simulink model "Torque Vectoring"  (R2023b)
settings: Solver=VariableStepAuto  StartTime=0.0  StopTime=10.0  RelTol=1e-3
model workspace (MAT data in the model file):
  Bx = 10
  By = 10
  Cd = 0.2
  Cx = 1.9
  Cy = 1.9
  Ex = 0.97
  Ey = 0.97
  Izz = 600
  Ki = 1
  Kp = 1
  Ku = 1
  Re = 0.25
  Ts = 0.01
  g = 9.8
  h = 0.3
  k = 100
  l = 2.25
  lf = 0.78
  lr = 0.78
  m = 300
  mu_x = 0.3
  mu_y = 0.2
  rho = 8
  s = 1
libraries: slpidlib x1
settings Model: Creator=Anand Chutani  LastModifiedBy=Anand Chutani
settings DebuggingCC: AlgebraicLoopMsg=none

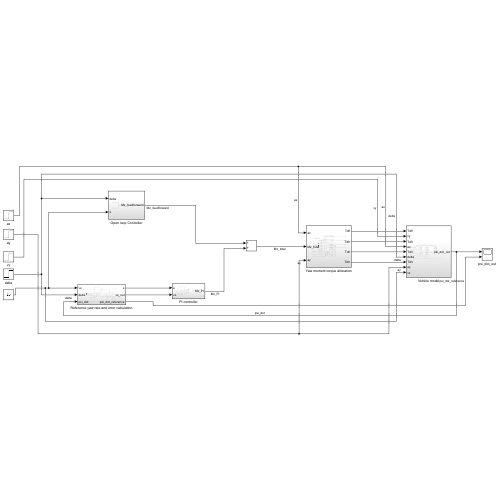
[thumbnail: Simulink's stored preview of the top-level diagram]
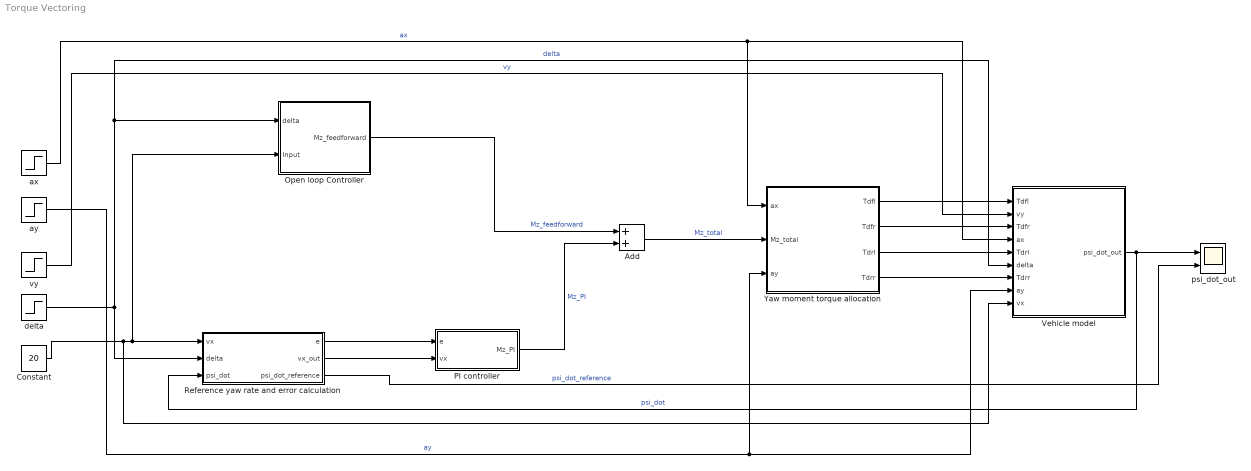
== system Torque Vectoring ==
  Add : Sum
  Constant : Constant  Value=20
  Open loop Controller : Subsystem
  PI controller : Subsystem
  Reference yaw rate and error calculation : Subsystem
  Vehicle model : Subsystem
  Yaw moment torque allocation : Subsystem
  ax : Step  Before=1  After=3  SampleTime=0
  ay : Step  Before=1  After=5  SampleTime=0
  delta : Step  Before=1  After=4  SampleTime=0
  psi_dot_out : Scope  NumInputPorts=2
  vy : Step  Before=12  After=14  SampleTime=0
  wires:
  Add/1 -> Yaw moment torque allocation/2(Mz_total)  "Mz_total"
  Yaw moment torque allocation/1(Tdfl) -> Vehicle model/1(Tdfl)
  Yaw moment torque allocation/2(Tdfr) -> Vehicle model/3(Tdfr)
  Yaw moment torque allocation/3(Tdrl) -> Vehicle model/5(Tdrl)
  Yaw moment torque allocation/4(Tdrr) -> Vehicle model/7(Tdrr)
  delta/1 -> Vehicle model/6(delta), Open loop Controller/1(delta), Reference yaw rate and error calculation/2(delta)  "delta"
  Vehicle model/1(psi_dot_out) -> Reference yaw rate and error calculation/3(psi_dot), psi_dot_out/1  "psi_dot"
  ax/1 -> Yaw moment torque allocation/1(ax), Vehicle model/4(ax)  "ax"
  ay/1 -> Yaw moment torque allocation/3(ay), Vehicle model/8(ay)  "ay"
  vy/1 -> Vehicle model/2(vy)  "vy"
  Reference yaw rate and error calculation/3(psi_dot_reference) -> psi_dot_out/2  "psi_dot_reference"
  Reference yaw rate and error calculation/1(e) -> PI controller/1(e)
  PI controller/1(Mz_PI) -> Add/2  "Mz_PI"
  Open loop Controller/1(Mz_feedforward) -> Add/1  "Mz_feedforward"
  Reference yaw rate and error calculation/2(vx_out) -> PI controller/2(vx)
  Constant/1 -> Vehicle model/9(vx), Open loop Controller/2(Input), Reference yaw rate and error calculation/1(vx)

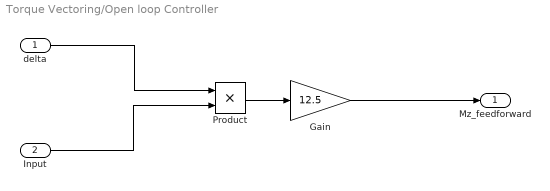
== system Torque Vectoring/Open loop Controller ==
  delta : Inport
  Input : Inport  Port=2
  Gain : Gain  Gain=12.5
  Product : Product
  Mz_feedforward : Outport
  wires:
  Gain/1 -> Mz_feedforward/1
  delta/1 -> Product/1
  Input/1 -> Product/2
  Product/1 -> Gain/1

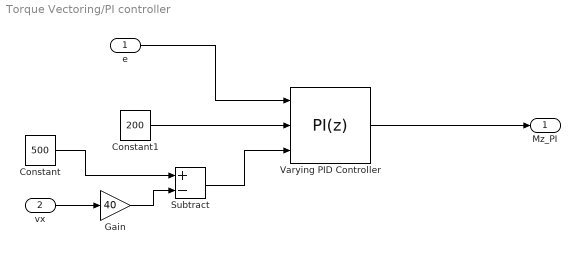
== system Torque Vectoring/PI controller ==
  e : Inport
  vx : Inport  Port=2
  Constant : Constant  Value=500
  Constant1 : Constant  Value=200
  Gain : Gain  Gain=40
  Subtract : Sum  Inputs=+-
  Varying PID Controller : slpidlib/PID Controller  Controller=PI  Form=Parallel  TimeDomain=Discrete-time  UseExternalTs=off  SampleTime=-1  IntegratorMethod=Forward Euler  FilterMethod=Forward Euler  ControllerParametersSource=external  P=1  I=1  UseKiTs=off  D=0  N=100  UseFilter=on  TunerSelectOption=Transfer Function Based (PID Tuner App)  InitialConditionSource=internal  InitialConditionForIntegrator=0  InitialConditionForFilter=0  DifferentiatorICPrevScaledInput=0  ExternalReset=none  TrackingMode=off  Kt=1  LimitOutput=off  SatLimitsSource=internal  UpperSaturationLimit=inf  LowerSaturationLimit=-inf  LinearizeAsGain=on  AntiWindupMode=none  Kb=1  LimitIntegrator=off  UpperIntegratorSaturationLimit=inf  LowerIntegratorSaturationLimit=-inf  POutMin=[]  POutMax=[]  IOutMin=[]  IOutMax=[]  DOutMin=[]  DOutMax=[]  NOutMin=[]  NOutMax=[]  SumOutMin=[]  SumOutMax=[]  SaturationOutMin=[]  SaturationOutMax=[]  PParamMin=[]  PParamMax=[]  IParamMin=[]  IParamMax=[]  DParamMin=[]  DParamMax=[]  NParamMin=[]  NParamMax=[]  KbParamMin=[]  KbParamMax=[]  KtParamMin=[]  KtParamMax=[]  KbOutMin=[]  KbOutMax=[]  KtOutMin=[]  KtOutMax=[]  IntegratorOutMin=[]  IntegratorOutMax=[]  FilterOutMin=[]  FilterOutMax=[]  SumI1OutMin=[]  SumI1OutMax=[]  SumI2OutMin=[]  SumI2OutMax=[]  SumI3OutMin=[]  SumI3OutMax=[]  SumI4OutMin=[]  SumI4OutMax=[]  SumDOutMin=[]  SumDOutMax=[]  DifferentiatorOutMin=[]  DifferentiatorOutMax=[]  FilterDiffOutCoefMin=[]  FilterDiffOutCoefMax=[]  ReciprocalOutMin=[]  ReciprocalOutMax=[]  SumDenOutMin=[]  SumDenOutMax=[]  SumNumOutMin=[]  SumNumOutMax=[]  DivideOutMin=[]  DivideOutMax=[]  UdiffTsProdOutMin=[]  UdiffTsProdOutMax=[]  NTsProdOutMin=[]  NTsProdOutMax=[]  UintegralTsProdOutMin=[]  UintegralTsProdOutMax=[]  UngainTsProdOutMin=[]  UngainTsProdOutMax=[]  ClampingZeroOutDataTypeStr=Inherit: Inherit via back propagation  ClampingZeroOutMin=[]  ClampingZeroOutMax=[]  FilterDenConstantOutDataTypeStr=Inherit: Inherit via back propagation  FilterDenConstantOutMin=[]  FilterDenConstantOutMax=[]  PCopyOutDataTypeStr=Inherit: Inherit via back propagation  PCopyOutMin=[]  PCopyOutMax=[]  NCopyOutDataTypeStr=Inherit: Inherit via back propagation  NCopyOutMin=[]  NCopyOutMax=[]  IntegratorContinuousStateAttributes=''  IntegratorStateMustResolveToSignalObject=off  IntegratorRTWStateStorageClass=Auto  FilterContinuousStateAttributes=''  FilterStateMustResolveToSignalObject=off  FilterRTWStateStorageClass=Auto  ParallelPVariant=ExternalParameters  IdealPVariant=Disabled  IVariant=ExternalParameters  DVariant=Disabled  IntegratorVariant=Discrete  SatVariant=Disabled  AWVariant=Passthrough  PCopyVariant=Disabled  TRVariant=Disabled  FdbkBlocksVariant=Forward  IdealPFdbkVariant=Disabled  SatFdbkVariant=Disabled  DerivativeFilterVariant=Disabled  NVariant=Disabled  NCopyVariant=Disabled_SignalSpec  FilterICVariant=Disabled  IntegratorICVariant=InternalICs  ExternalResetVariant=Disabled  TRSumVariant=Passthrough  SumFdbkVariant=Disabled  SumVariant=Sum_PI  TsampFilterVariant=InternalTs  TsampNgainVariant=Passthrough  TsampIntegralVariant=Disabled_SignalSpec  ExternalSaturationOutDataTypeStr=Inherit: Same as second input
      settings: LibrarySourceBlock=cstblocks/Linear Parameter Varying/Varying PID Controller
  Mz_PI : Outport
  wires:
  Varying PID Controller/1 -> Mz_PI/1
  vx/1 -> Gain/1
  e/1 -> Varying PID Controller/1
  Constant/1 -> Subtract/1
  Subtract/1 -> Varying PID Controller/3
  Constant1/1 -> Varying PID Controller/2
  Gain/1 -> Subtract/2

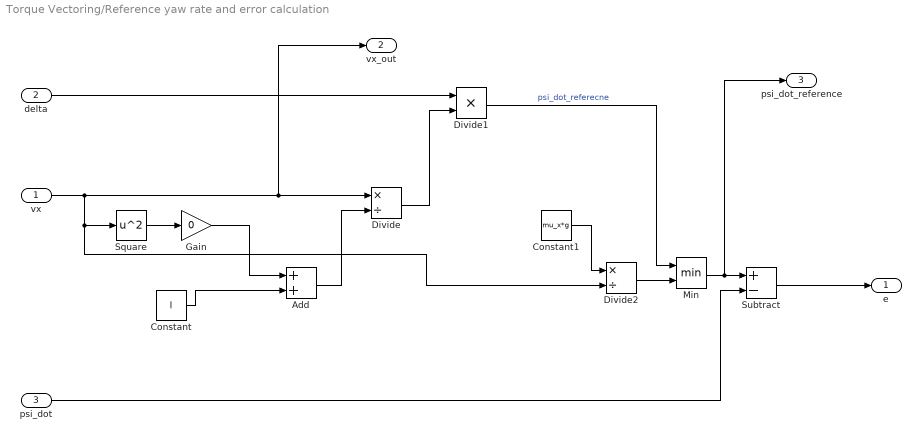
== system Torque Vectoring/Reference yaw rate and error calculation ==
  vx : Inport
  delta : Inport  Port=2
  psi_dot : Inport  Port=3
  Add : Sum
  Constant : Constant  Value=l
  Constant1 : Constant  Value=mu_x*g
  Divide : Product  Inputs=*/
  Divide1 : Product  Inputs=**
  Divide2 : Product  Inputs=*/
  Gain : Gain  Gain=0
  Min : MinMax  Inputs=2
  Square : Math  Operator=square
  Subtract : Sum  Inputs=+-
  e : Outport
  vx_out : Outport  Port=2
  psi_dot_reference : Outport  Port=3
  wires:
  vx/1 -> vx_out/1, Divide/1, Divide2/2, Square/1
  Square/1 -> Gain/1
  Gain/1 -> Add/1
  Constant/1 -> Add/2
  Add/1 -> Divide/2
  delta/1 -> Divide1/1
  Divide/1 -> Divide1/2
  Divide1/1 -> Min/1  "psi_dot_referecne"
  psi_dot/1 -> Subtract/2
  Subtract/1 -> e/1
  Constant1/1 -> Divide2/1
  Divide2/1 -> Min/2
  Min/1 -> psi_dot_reference/1, Subtract/1

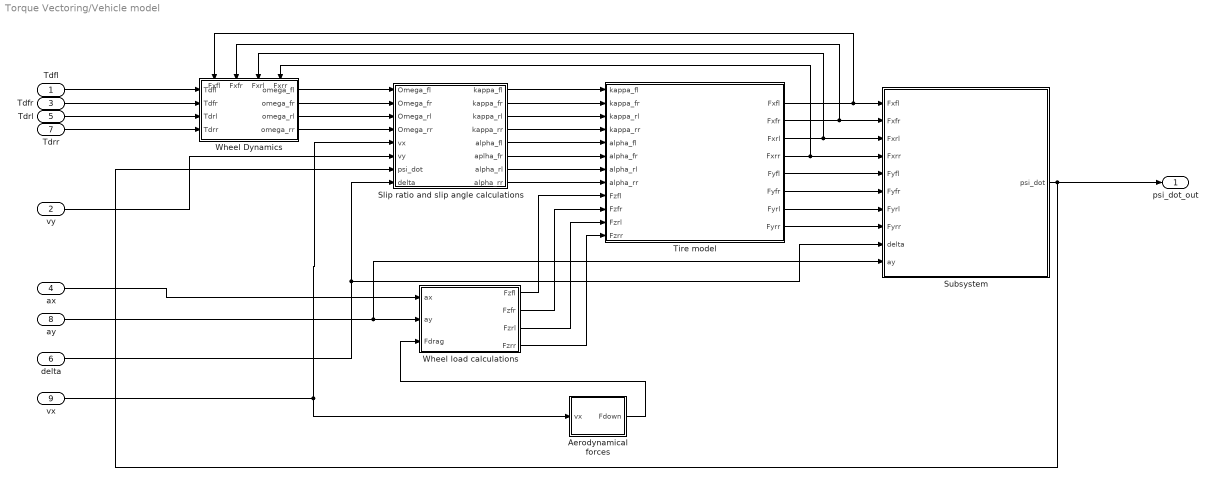
== system Torque Vectoring/Vehicle model ==
  Tdfl : Inport
  vy : Inport  Port=2
  Tdfr : Inport  Port=3
  ax : Inport  Port=4
  Tdrl : Inport  Port=5
  delta : Inport  Port=6
  Tdrr : Inport  Port=7
  ay : Inport  Port=8
  vx : Inport  Port=9
  Aerodynamical forces : Subsystem
  Slip ratio and slip angle calculations : Subsystem
  Subsystem : Subsystem
  Tire model : Subsystem
  Wheel Dynamics : Subsystem
      settings: PortSchema="{\"entries\":[{\"content\":{\"sides\":[{\"content\":{\"connectorIds\":[\"In1\",\"In2\",\"In3\",\"In4\"]},\"type\":\"ConnectorPlacement.EquallySpacedRectSide\",\"uuid\":\"cf3d01e9-74dd-45bb-b04b-f5977a1fd43e\"},{\"content\":{\"connectorIds\":[\"Out1\",\"Out2\",\"Out3\",\"Out4\"],\"side\":\"RIGHT\"},\"type\":\"ConnectorPlacement.EquallySpacedRectSide\",\"uuid\":\"48e33519-fc03-4ace-b300-f3df5174e3b2\"},{\"content\":{\"connectorIds\":[\"In5\",\"In6\",\"In7\",\"In8\"],\"side\":\"TOP\"},\"type\":\"ConnectorPlacement.EquallySpacedRectSide\",\"uuid\":\"343d2f22-4e97-404d-bc1a-e31503635e2d\"}]},\"type\":\"ConnectorPlacement.EquallySpacedConnector\",\"uuid\":\"a3e340ec-438c-437e-9241-e2a33ee22be6\"}],\"packageUris\":[\"http://schema.mathworks.com/mf0/Connector/R2020b\"],\"version\":\"1.0\"}"
  Wheel load calculations : Subsystem
  psi_dot_out : Outport
  wires:
  Wheel Dynamics/1(omega_fl) -> Slip ratio and slip angle calculations/1(Omega_fl)
  Wheel Dynamics/2(omega_fr) -> Slip ratio and slip angle calculations/2(Omega_fr)
  Wheel Dynamics/3(omega_rl) -> Slip ratio and slip angle calculations/3(Omega_rl)
  Wheel Dynamics/4(omega_rr) -> Slip ratio and slip angle calculations/4(Omega_rr)
  vy/1 -> Slip ratio and slip angle calculations/6(vy)
  delta/1 -> Slip ratio and slip angle calculations/8(delta), Subsystem/9(delta)
  Aerodynamical forces/1(Fdown) -> Wheel load calculations/3(Fdrag)
  Slip ratio and slip angle calculations/1(kappa_fl) -> Tire model/1(kappa_fl)
  Slip ratio and slip angle calculations/2(kappa_fr) -> Tire model/2(kappa_fr)
  Slip ratio and slip angle calculations/3(kappa_rl) -> Tire model/3(kappa_rl)
  Slip ratio and slip angle calculations/4(kappa_rr) -> Tire model/4(kappa_rr)
  Slip ratio and slip angle calculations/5(alpha_fl) -> Tire model/5(alpha_fl)
  Slip ratio and slip angle calculations/6(aplha_fr) -> Tire model/6(alpha_fr)
  Slip ratio and slip angle calculations/7(alpha_rl) -> Tire model/7(alpha_rl)
  Slip ratio and slip angle calculations/8(alpha_rr) -> Tire model/8(alpha_rr)
  Wheel load calculations/1(Fzfl) -> Tire model/9(Fzfl)
  Wheel load calculations/2(Fzfr) -> Tire model/10(Fzfr)
  Wheel load calculations/3(Fzrl) -> Tire model/11(Fzrl)
  Wheel load calculations/4(Fzrr) -> Tire model/12(Fzrr)
  Tire model/1(Fxfl) -> Wheel Dynamics/5(Fxfl), Subsystem/1(Fxfl)
  Tire model/2(Fxfr) -> Subsystem/2(Fxfr), Wheel Dynamics/6(Fxfr)
  Tire model/3(Fxrl) -> Wheel Dynamics/7(Fxrl), Subsystem/3(Fxrl)
  Tire model/4(Fxrr) -> Subsystem/4(Fxrr), Wheel Dynamics/8(Fxrr)
  Tire model/5(Fyfl) -> Subsystem/5(Fyfl)
  Tire model/6(Fyfr) -> Subsystem/6(Fyfr)
  Tire model/7(Fyrl) -> Subsystem/7(Fyrl)
  Tire model/8(Fyrr) -> Subsystem/8(Fyrr)
  ay/1 -> Wheel load calculations/2(ay), Subsystem/10(ay)
  ax/1 -> Wheel load calculations/1(ax)
  Subsystem/1(psi_dot) -> psi_dot_out/1, Slip ratio and slip angle calculations/7(psi_dot)
  Tdfl/1 -> Wheel Dynamics/1(Tdfl)
  Tdfr/1 -> Wheel Dynamics/2(Tdfr)
  Tdrl/1 -> Wheel Dynamics/3(Tdrl)
  Tdrr/1 -> Wheel Dynamics/4(Tdrr)
  vx/1 -> Slip ratio and slip angle calculations/5(vx), Aerodynamical forces/1(vx)

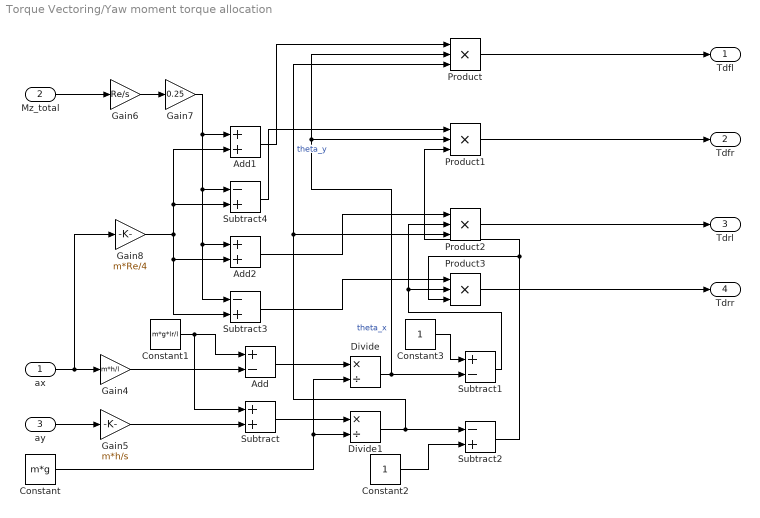
== system Torque Vectoring/Yaw moment torque allocation ==
  ax : Inport
  Mz_total : Inport  Port=2
  ay : Inport  Port=3
  Add : Sum  Inputs=+-
  Add1 : Sum
  Add2 : Sum
  Constant : Constant  Value=m*g
  Constant1 : Constant  Value=m*g*lr/l
  Constant2 : Constant
  Constant3 : Constant
  Divide : Product  Inputs=*/
  Divide1 : Product  Inputs=*/
  Gain4 : Gain  Gain=m*h/l
  Gain5 : Gain  Gain=m*h/s
  Gain6 : Gain  Gain=Re/s
  Gain7 : Gain  Gain=0.25
  Gain8 : Gain  Gain=m*Re/4
  Product{,1..3} (4 alike) : Product  Inputs=3
  Subtract : Sum
  Subtract1 : Sum  Inputs=+-
  Subtract2 : Sum  Inputs=-+
  Subtract3 : Sum  Inputs=-+
  Subtract4 : Sum  Inputs=-+
  Tdfl : Outport
  Tdfr : Outport  Port=2
  Tdrl : Outport  Port=3
  Tdrr : Outport  Port=4
  wires:
  ax/1 -> Gain8/1, Gain4/1
  ay/1 -> Gain5/1
  Constant1/1 -> Subtract/1, Add/1
  Gain4/1 -> Add/2
  Add/1 -> Divide/1
  Constant/1 -> Divide1/2, Divide/2
  Divide/1 -> Subtract1/2, Product1/2, Product/2  "theta_x"
  Gain5/1 -> Subtract/2
  Subtract/1 -> Divide1/1
  Divide1/1 -> Subtract2/1, Product/3, Product2/3  "theta_y"
  Constant2/1 -> Subtract2/2
  Constant3/1 -> Subtract1/1
  Subtract2/1 -> Product1/3, Product3/3
  Subtract1/1 -> Product3/2, Product2/2
  Mz_total/1 -> Gain6/1
  Gain6/1 -> Gain7/1
  Gain7/1 -> Subtract4/1, Subtract3/1, Add2/1, Add1/1
  Add1/1 -> Product/1
  Subtract4/1 -> Product1/1
  Add2/1 -> Product2/1
  Subtract3/1 -> Product3/1
  Product/1 -> Tdfl/1
  Product1/1 -> Tdfr/1
  Product2/1 -> Tdrl/1
  Product3/1 -> Tdrr/1
  Gain8/1 -> Subtract3/2, Add2/2, Subtract4/2, Add1/2

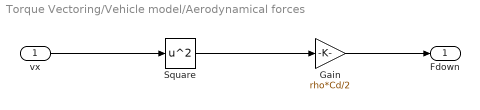
== system Torque Vectoring/Vehicle model/Aerodynamical forces ==
  vx : Inport
  Gain : Gain  Gain=rho*Cd/2
  Square : Math  Operator=square
  Fdown : Outport
  wires:
  vx/1 -> Square/1
  Gain/1 -> Fdown/1
  Square/1 -> Gain/1

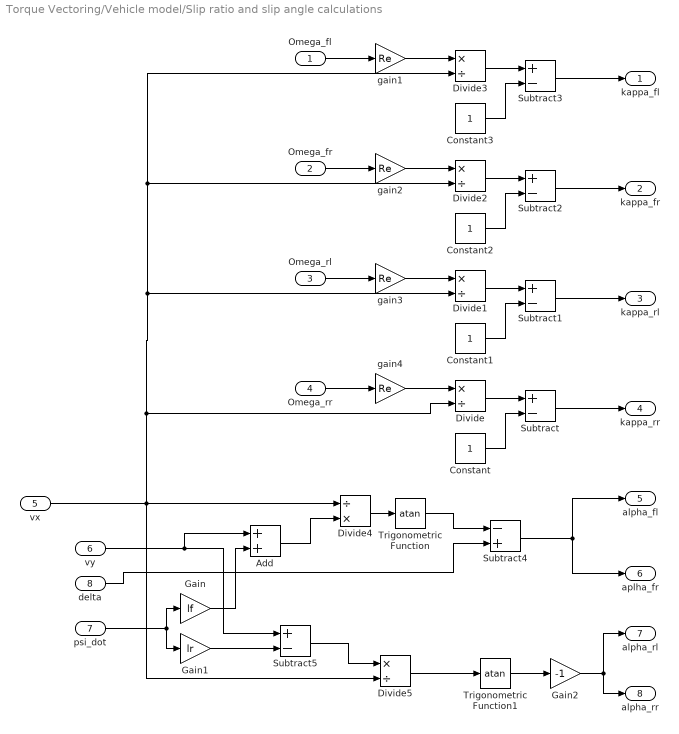
== system Torque Vectoring/Vehicle model/Slip ratio and slip angle calculations ==
  Omega_fl : Inport
  Omega_fr : Inport  Port=2
  Omega_rl : Inport  Port=3
  Omega_rr : Inport  Port=4
  vx : Inport  Port=5
  vy : Inport  Port=6
  psi_dot : Inport  Port=7
  delta : Inport  Port=8
  Add : Sum
  Constant{,1..3} (4 alike) : Constant
  Divide{,1..3,5} (5 alike) : Product  Inputs=*/
  Divide4 : Product  Inputs=/*
  Gain : Gain  Gain=lf
  Gain1 : Gain  Gain=lr
  Gain2 : Gain  Gain=-1
  Subtract{,1..3,5} (5 alike) : Sum  Inputs=+-
  Subtract4 : Sum  Inputs=-+
  Trigonometric Function : Trigonometry  Operator=atan
  Trigonometric Function1 : Trigonometry  Operator=atan
  gain{1..4} (4 alike) : Gain  Gain=Re
  kappa_fl : Outport
  kappa_fr : Outport  Port=2
  kappa_rl : Outport  Port=3
  kappa_rr : Outport  Port=4
  alpha_fl : Outport  Port=5
  aplha_fr : Outport  Port=6
  alpha_rl : Outport  Port=7
  alpha_rr : Outport  Port=8
  wires:
  Omega_rr/1 -> gain4/1
  gain4/1 -> Divide/1
  Divide/1 -> Subtract/1
  Constant/1 -> Subtract/2
  Subtract/1 -> kappa_rr/1
  Subtract1/1 -> kappa_rl/1
  gain3/1 -> Divide1/1
  Constant1/1 -> Subtract1/2
  Omega_rl/1 -> gain3/1
  Divide1/1 -> Subtract1/1
  Subtract2/1 -> kappa_fr/1
  gain2/1 -> Divide2/1
  Constant2/1 -> Subtract2/2
  Omega_fr/1 -> gain2/1
  Divide2/1 -> Subtract2/1
  Subtract3/1 -> kappa_fl/1
  gain1/1 -> Divide3/1
  Constant3/1 -> Subtract3/2
  Omega_fl/1 -> gain1/1
  Divide3/1 -> Subtract3/1
  vy/1 -> Subtract5/1, Add/1
  psi_dot/1 -> Gain1/1, Gain/1
  Gain/1 -> Add/2
  Add/1 -> Divide4/2
  Divide4/1 -> Trigonometric Function/1
  delta/1 -> Subtract4/2
  Trigonometric Function/1 -> Subtract4/1
  Subtract4/1 -> aplha_fr/1, alpha_fl/1
  Gain1/1 -> Subtract5/2
  Subtract5/1 -> Divide5/1
  Trigonometric Function1/1 -> Gain2/1
  Gain2/1 -> alpha_rr/1, alpha_rl/1
  Divide5/1 -> Trigonometric Function1/1
  vx/1 -> Divide3/2, Divide2/2, Divide1/2, Divide/2, Divide4/1, Divide5/2

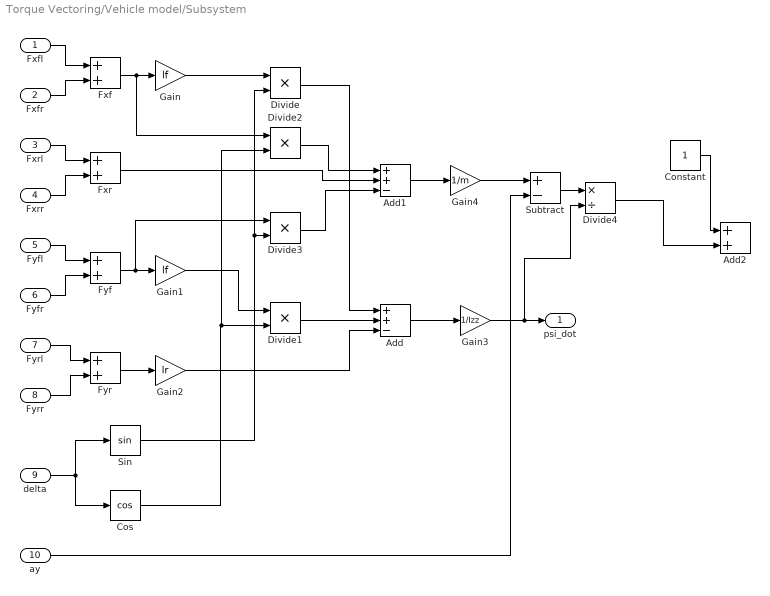
== system Torque Vectoring/Vehicle model/Subsystem ==
  Fxfl : Inport
  Fxfr : Inport  Port=2
  Fxrl : Inport  Port=3
  Fxrr : Inport  Port=4
  Fyfl : Inport  Port=5
  Fyfr : Inport  Port=6
  Fyrl : Inport  Port=7
  Fyrr : Inport  Port=8
  delta : Inport  Port=9
  ay : Inport  Port=10
  Add : Sum  Inputs=++-
  Add1 : Sum  Inputs=++-
  Add2 : Sum
  Constant : Constant
  Cos : Trigonometry  Operator=cos
  Divide{,1..3} (4 alike) : Product  Inputs=**
  Divide4 : Product  Inputs=*/
  Fxf : Sum
  Fxr : Sum
  Fyf : Sum
  Fyr : Sum
  Gain : Gain  Gain=lf
  Gain1 : Gain  Gain=lf
  Gain2 : Gain  Gain=lr
  Gain3 : Gain  Gain=1/Izz
  Gain4 : Gain  Gain=1/m
  Sin : Trigonometry
  Subtract : Sum  Inputs=+-
  psi_dot : Outport
  wires:
  Fxfl/1 -> Fxf/1
  Fxfr/1 -> Fxf/2
  Fxrl/1 -> Fxr/1
  Fxrr/1 -> Fxr/2
  Fyfl/1 -> Fyf/1
  Fyfr/1 -> Fyf/2
  Fyrl/1 -> Fyr/1
  Fyrr/1 -> Fyr/2
  Fxf/1 -> Divide2/1, Gain/1
  delta/1 -> Cos/1, Sin/1
  Sin/1 -> Divide3/2, Divide/2
  Gain/1 -> Divide/1
  Fyf/1 -> Divide3/1, Gain1/1
  Gain1/1 -> Divide1/1
  Cos/1 -> Divide2/2, Divide1/2
  Fyr/1 -> Gain2/1
  Divide/1 -> Add/1
  Divide1/1 -> Add/2
  Gain2/1 -> Add/3
  Add/1 -> Gain3/1
  Gain3/1 -> Divide4/2, psi_dot/1
  Divide2/1 -> Add1/1
  Fxr/1 -> Add1/2
  Divide3/1 -> Add1/3
  Add1/1 -> Gain4/1
  Gain4/1 -> Subtract/1
  ay/1 -> Subtract/2
  Subtract/1 -> Divide4/1
  Divide4/1 -> Add2/2
  Constant/1 -> Add2/1

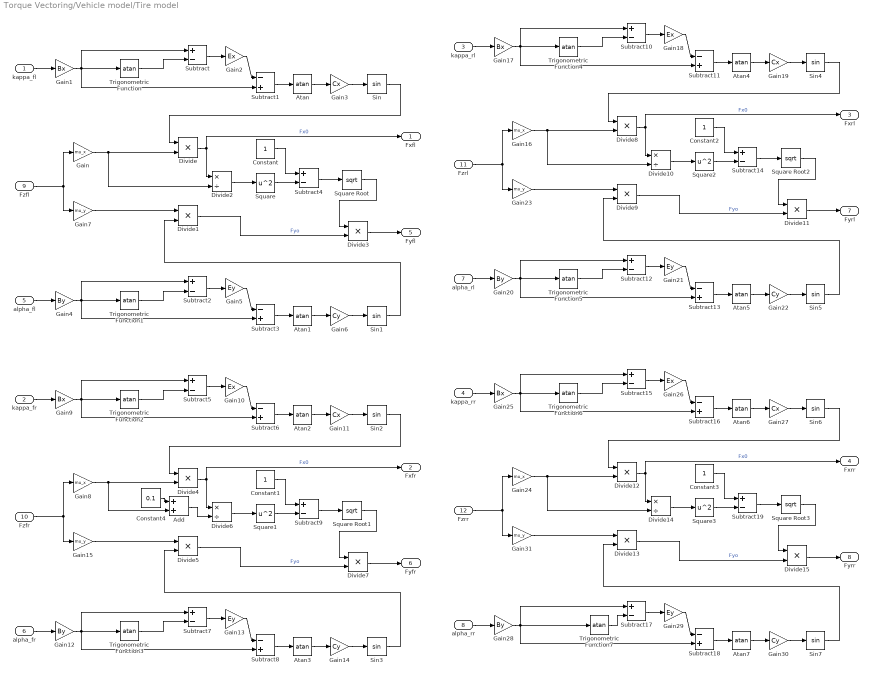
== system Torque Vectoring/Vehicle model/Tire model ==
  kappa_fl : Inport
  kappa_fr : Inport  Port=2
  kappa_rl : Inport  Port=3
  kappa_rr : Inport  Port=4
  alpha_fl : Inport  Port=5
  alpha_fr : Inport  Port=6
  alpha_rl : Inport  Port=7
  alpha_rr : Inport  Port=8
  Fzfl : Inport  Port=9
  Fzfr : Inport  Port=10
  Fzrl : Inport  Port=11
  Fzrr : Inport  Port=12
  Add : Sum
  Atan{,1..7} (8 alike) : Trigonometry  Operator=atan
  Constant{,1..3} (4 alike) : Constant
  Constant4 : Constant  Value=0.1
  Divide{,1,3..5,7..9,11..13,15} (12 alike) : Product  Inputs=**
  Divide{2,6,10,14} (4 alike) : Product  Inputs=*/
  Gain{,8,16,24} (4 alike) : Gain  Gain=mu_x
  Gain{1,9,17,25} (4 alike) : Gain  Gain=Bx
  Gain{2,10,18,26} (4 alike) : Gain  Gain=Ex
  Gain{3,11,19,27} (4 alike) : Gain  Gain=Cx
  Gain{4,12,20,28} (4 alike) : Gain  Gain=By
  Gain{5,13,21,29} (4 alike) : Gain  Gain=Ey
  Gain{6,14,22,30} (4 alike) : Gain  Gain=Cy
  Gain{7,15,23,31} (4 alike) : Gain  Gain=mu_y
  Sin{,1..7} (8 alike) : Trigonometry
  Square{,1..3} (4 alike) : Math  Operator=square
  Square Root{,1..3} (4 alike) : Sqrt
  Subtract{,2,4..5,7,9..10,12,14..15,17,19} (12 alike) : Sum  Inputs=+-
  Subtract{1,3,6,8,11,13,16,18} (8 alike) : Sum  Inputs=-+
  Trigonometric Function{,1..7} (8 alike) : Trigonometry  Operator=atan
  Fxfl : Outport
  Fxfr : Outport  Port=2
  Fxrl : Outport  Port=3
  Fxrr : Outport  Port=4
  Fyfl : Outport  Port=5
  Fyfr : Outport  Port=6
  Fyrl : Outport  Port=7
  Fyrr : Outport  Port=8
  wires:
  Fzfl/1 -> Gain7/1, Gain/1
  kappa_fl/1 -> Gain1/1
  Gain1/1 -> Subtract1/2, Trigonometric Function/1, Subtract/1
  Trigonometric Function/1 -> Subtract/2
  Subtract/1 -> Gain2/1
  Gain2/1 -> Subtract1/1
  Subtract1/1 -> Atan/1
  Atan/1 -> Gain3/1
  Gain3/1 -> Sin/1
  Gain/1 -> Divide2/2, Divide/2
  Sin/1 -> Divide/1
  Divide/1 -> Divide2/1, Fxfl/1  "Fx0"
  Trigonometric Function1/1 -> Subtract2/2
  Gain4/1 -> Subtract3/2, Trigonometric Function1/1, Subtract2/1
  Subtract3/1 -> Atan1/1
  Atan1/1 -> Gain6/1
  Subtract2/1 -> Gain5/1
  alpha_fl/1 -> Gain4/1
  Gain5/1 -> Subtract3/1
  Gain6/1 -> Sin1/1
  Sin1/1 -> Divide1/2
  Gain7/1 -> Divide1/1
  Divide1/1 -> Divide3/2  "Fyo"
  Divide2/1 -> Square/1
  Constant/1 -> Subtract4/1
  Square/1 -> Subtract4/2
  Subtract4/1 -> Square Root/1
  Square Root/1 -> Divide3/1
  Divide3/1 -> Fyfl/1
  Divide4/1 -> Divide6/1, Fxfr/1  "Fx0"
  Trigonometric Function2/1 -> Subtract5/2
  Constant1/1 -> Subtract9/1
  Divide6/1 -> Square1/1
  Gain8/1 -> Add/2, Divide4/2
  Sin2/1 -> Divide4/1
  Gain11/1 -> Sin2/1
  kappa_fr/1 -> Gain9/1
  Subtract9/1 -> Square Root1/1
  Fzfr/1 -> Gain15/1, Gain8/1
  Subtract6/1 -> Atan2/1
  Divide7/1 -> Fyfr/1
  alpha_fr/1 -> Gain12/1
  Divide5/1 -> Divide7/2  "Fyo"
  Sin3/1 -> Divide5/2
  Atan2/1 -> Gain11/1
  Gain15/1 -> Divide5/1
  Gain9/1 -> Subtract6/2, Trigonometric Function2/1, Subtract5/1
  Square Root1/1 -> Divide7/1
  Subtract5/1 -> Gain10/1
  Gain13/1 -> Subtract8/1
  Atan3/1 -> Gain14/1
  Square1/1 -> Subtract9/2
  Subtract8/1 -> Atan3/1
  Gain14/1 -> Sin3/1
  Gain12/1 -> Subtract8/2, Trigonometric Function3/1, Subtract7/1
  Subtract7/1 -> Gain13/1
  Gain10/1 -> Subtract6/1
  Trigonometric Function3/1 -> Subtract7/2
  Divide8/1 -> Divide10/1, Fxrl/1  "Fx0"
  Trigonometric Function4/1 -> Subtract10/2
  Constant2/1 -> Subtract14/1
  Divide10/1 -> Square2/1
  Gain16/1 -> Divide10/2, Divide8/2
  Sin4/1 -> Divide8/1
  Gain19/1 -> Sin4/1
  kappa_rl/1 -> Gain17/1
  Subtract14/1 -> Square Root2/1
  Fzrl/1 -> Gain23/1, Gain16/1
  Subtract11/1 -> Atan4/1
  Divide11/1 -> Fyrl/1
  alpha_rl/1 -> Gain20/1
  Divide9/1 -> Divide11/2  "Fyo"
  Sin5/1 -> Divide9/2
  Atan4/1 -> Gain19/1
  Gain23/1 -> Divide9/1
  Gain17/1 -> Subtract11/2, Trigonometric Function4/1, Subtract10/1
  Square Root2/1 -> Divide11/1
  Subtract10/1 -> Gain18/1
  Gain21/1 -> Subtract13/1
  Atan5/1 -> Gain22/1
  Square2/1 -> Subtract14/2
  Subtract13/1 -> Atan5/1
  Gain22/1 -> Sin5/1
  Gain20/1 -> Subtract13/2, Trigonometric Function5/1, Subtract12/1
  Subtract12/1 -> Gain21/1
  Gain18/1 -> Subtract11/1
  Trigonometric Function5/1 -> Subtract12/2
  Divide12/1 -> Divide14/1, Fxrr/1  "Fx0"
  Trigonometric Function6/1 -> Subtract15/2
  Constant3/1 -> Subtract19/1
  Divide14/1 -> Square3/1
  Gain24/1 -> Divide14/2, Divide12/2
  Sin6/1 -> Divide12/1
  Gain27/1 -> Sin6/1
  kappa_rr/1 -> Gain25/1
  Subtract19/1 -> Square Root3/1
  Fzrr/1 -> Gain31/1, Gain24/1
  Subtract16/1 -> Atan6/1
  Divide15/1 -> Fyrr/1
  alpha_rr/1 -> Gain28/1
  Divide13/1 -> Divide15/2  "Fyo"
  Sin7/1 -> Divide13/2
  Atan6/1 -> Gain27/1
  Gain31/1 -> Divide13/1
  Gain25/1 -> Subtract16/2, Trigonometric Function6/1, Subtract15/1
  Square Root3/1 -> Divide15/1
  Subtract15/1 -> Gain26/1
  Gain29/1 -> Subtract18/1
  Atan7/1 -> Gain30/1
  Square3/1 -> Subtract19/2
  Subtract18/1 -> Atan7/1
  Gain30/1 -> Sin7/1
  Gain28/1 -> Subtract18/2, Trigonometric Function7/1, Subtract17/1
  Subtract17/1 -> Gain29/1
  Gain26/1 -> Subtract16/1
  Trigonometric Function7/1 -> Subtract17/2
  Constant4/1 -> Add/1
  Add/1 -> Divide6/2

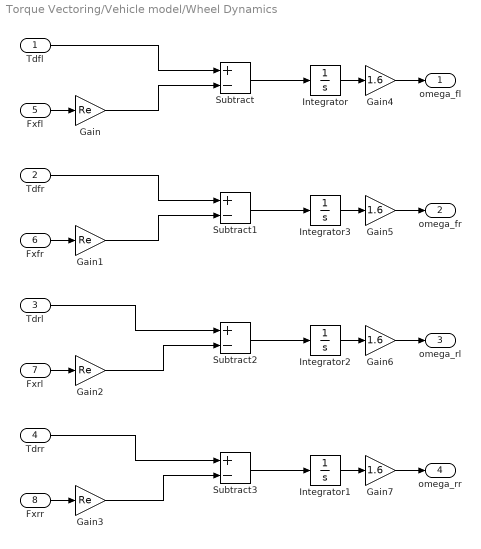
== system Torque Vectoring/Vehicle model/Wheel Dynamics ==
  Tdfl : Inport
  Tdfr : Inport  Port=2
  Tdrl : Inport  Port=3
  Tdrr : Inport  Port=4
  Fxfl : Inport  Port=5
  Fxfr : Inport  Port=6
  Fxrl : Inport  Port=7
  Fxrr : Inport  Port=8
  Gain{,1..3} (4 alike) : Gain  Gain=Re
  Gain{4..7} (4 alike) : Gain  Gain=1.6
  Integrator{,1..3} (4 alike) : Integrator
  Subtract{,1..3} (4 alike) : Sum  Inputs=+-
  omega_fl : Outport
  omega_fr : Outport  Port=2
  omega_rl : Outport  Port=3
  omega_rr : Outport  Port=4
  wires:
  Fxfl/1 -> Gain/1
  Fxfr/1 -> Gain1/1
  Fxrl/1 -> Gain2/1
  Fxrr/1 -> Gain3/1
  Tdfl/1 -> Subtract/1
  Gain/1 -> Subtract/2
  Tdfr/1 -> Subtract1/1
  Gain1/1 -> Subtract1/2
  Tdrl/1 -> Subtract2/1
  Gain2/1 -> Subtract2/2
  Tdrr/1 -> Subtract3/1
  Gain3/1 -> Subtract3/2
  Subtract/1 -> Integrator/1
  Integrator/1 -> Gain4/1
  Subtract1/1 -> Integrator3/1
  Subtract2/1 -> Integrator2/1
  Subtract3/1 -> Integrator1/1
  Integrator3/1 -> Gain5/1
  Integrator2/1 -> Gain6/1
  Integrator1/1 -> Gain7/1
  Gain7/1 -> omega_rr/1
  Gain6/1 -> omega_rl/1
  Gain5/1 -> omega_fr/1
  Gain4/1 -> omega_fl/1

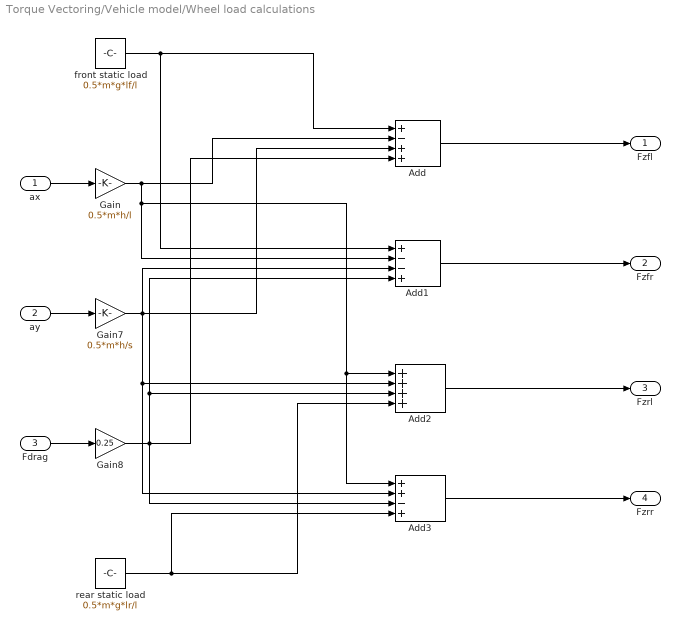
== system Torque Vectoring/Vehicle model/Wheel load calculations ==
  ax : Inport
  ay : Inport  Port=2
  Fdrag : Inport  Port=3
  Add : Sum  Inputs=+-++
  Add1 : Sum  Inputs=+--+
  Add2 : Sum  Inputs=++++
  Add3 : Sum  Inputs=++-+
  Gain : Gain  Gain=0.5*m*h/l
  Gain7 : Gain  Gain=0.5*m*h/s
  Gain8 : Gain  Gain=0.25
  front static load : Constant  Value=0.5*m*g*lf/l
  rear static load : Constant  Value=0.5*m*g*lr/l
  Fzfl : Outport
  Fzfr : Outport  Port=2
  Fzrl : Outport  Port=3
  Fzrr : Outport  Port=4
  wires:
  ax/1 -> Gain/1
  Fdrag/1 -> Gain8/1
  ay/1 -> Gain7/1
  front static load/1 -> Add1/1, Add/1
  Gain/1 -> Add3/1, Add2/1, Add1/2, Add/2
  Gain7/1 -> Add3/2, Add2/2, Add1/3, Add/3
  Gain8/1 -> Add3/3, Add1/4, Add2/3, Add/4
  Add/1 -> Fzfl/1
  Add1/1 -> Fzfr/1
  Add2/1 -> Fzrl/1
  rear static load/1 -> Add3/4, Add2/4
  Add3/1 -> Fzrr/1
